simulink model "usb_servo_wzorzec"  (R2015a)
settings: Solver=ode4  StartTime=0.0  StopTime=300  FixedStep=0.01  RelTol=1e-3
Description:
  | Real-Time Van der Pol Simulation
  | 
  | This demonstration shows a real-time version of the Simulink Van der Pol
  | simulation demo. This model does not need any external signals, so it does
  | not need any data acquisition hardware or driver. This makes the model ideal
  | for first experiments with Real-Time Windows Target, without need to
  | worry about proper I/O hardware configuration.
  | 
  | How to run this demo:
  | 
  |   1. Build the model using Tools -> Real-Time Workshop -> Build Model.
  |   2. Connect to the real-time code using Simulation -> Connect to target.
  |   3. Start the real-time execution using Simulation -> Start real-time code.
settings Model: SimulationMode=external  CovSFcnEnable=off  ExtModeTrigDuration=6000  Creator=Houska  LastModifiedBy=Student
settings DataIOCC: SignalLoggingSaveFormat=ModelDataLogs  SaveOutput=off  SaveTime=off  SignalLoggingName=logsOut
settings OptimizationCC: ExpressionDepthLimit=2147483647  InitFltsAndDblsToZero=on
settings DebuggingCC: SaveWithParameterizedLinksMsg=none  UnderspecifiedInitializationDetection=Classic  MergeDetectMultiDrivingBlocksExec=none  SignalResolutionControl=TryResolveAllWithWarning  MultiTaskDSMMsg=warning  MultiTaskCondExecSysMsg=none  FcnCallInpInsideContextMsg=UseLocalSettings  StateNameClashWarn=warning
settings HardwareCC: ProdIntDivRoundTo=Zero  ProdEndianess=LittleEndian  ProdHWDeviceType=32-bit Real-Time Windows Target  TargetHWDeviceType=32-bit Generic  ProdEqTarget=off
settings RTWCC: SystemTargetFile=rtcon_servo_usb2.tlc  TemplateMakefile=servo_vc_usb2_x64.tmf  Description=servo (Visual C/C++)
settings STFCustomTargetCC: GenerateSampleERTMain=off  ModelReferenceCompliant=off  GeneratePreprocessorConditionals=Disable all  CombineOutputUpdateFcns=on  ERTCustomFileBanners=off  MatFileLogging=on  SupportNonInlinedSFcns=on  SupportVariableSizeSignals=off  MATLABClassNameForMDSCustomization=Simulink.SoftwareTarget.GRTCustomization  SystemTargetFile=rtcon_servo_usb2.tlc
settings GRTTargetCC: ModelReferenceCompliant=off  ParMdlRefBuildCompliant=off  CompOptLevelCompliant=off  ConcurrentExecutionCompliant=off  CPPClassGenCompliant=off  ExtMode=on  ExtModeMexFile=rtcon_ext_comm

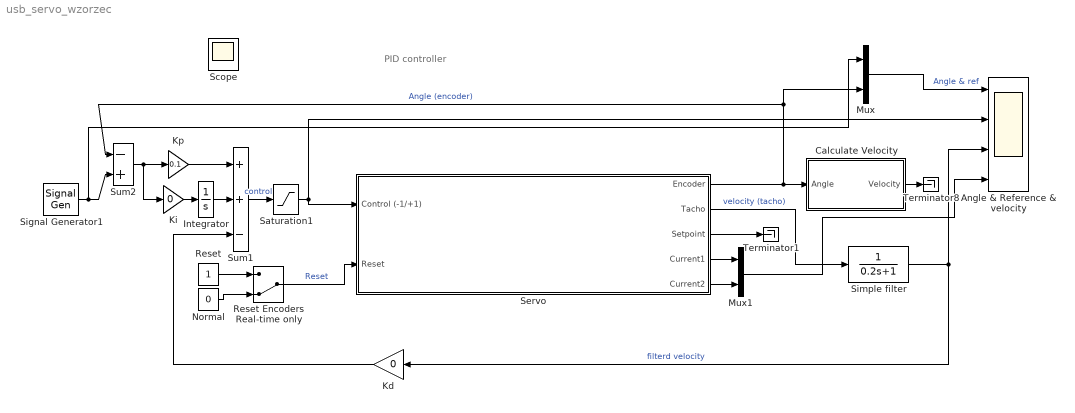
== system usb_servo_wzorzec ==
  note: PID controller
  Angle & Reference & velocity : Scope  NumInputPorts=4
      settings: TimeRange=30  YMin=-50~-0.6~-25~-10  YMax=60~0.6~45~8  SaveName=PD_C  MaxDataPoints=20000  Decimation=2
  Calculate Velocity : Subsystem
      mask Display: disp( 'rad-to-rad/s' )
  Integrator : Integrator
  Kd : Gain  Gain=0  SaturateOnIntegerOverflow=on  OutDataTypeStr=Inherit: Same as input  ParamDataTypeStr=Inherit: Same as input
  Ki : Gain  Gain=0  SaturateOnIntegerOverflow=on  OutDataTypeStr=Inherit: Same as input  ParamDataTypeStr=Inherit: Same as input
  Kp : Gain  Gain=0.1  SaturateOnIntegerOverflow=on  OutDataTypeStr=Inherit: Same as input  ParamDataTypeStr=Inherit: Same as input
  Mux : Mux  Inputs=2
  Mux1 : Mux  Inputs=2
  Normal : Constant  Value=0
  Reset : Constant
  Reset Encoders Real-time only : ManualSwitch  CurrentSetting=0
  Saturation1 : Saturate  UpperLimit=0.6  LowerLimit=-0.6
  Servo : Subsystem
      mask Display: image(imread('Servo.JPG'))
  Signal Generator1 : SignalGenerator  WaveForm=square  Amplitude=pi*25/2  Frequency=0.05
  Simple filter : TransferFcn  Denominator=[0.2 1]
  Sum1 : Sum  Inputs=++-  SaturateOnIntegerOverflow=on  InputSameDT=on  OutDataTypeStr=Inherit: Same as first input
  Sum2 : Sum  Inputs=-+  SaturateOnIntegerOverflow=on  InputSameDT=on  OutDataTypeStr=Inherit: Same as first input
  Terminator1 : Terminator
  Terminator8 : Terminator
  Scope : Scope
      settings: YMin=-5850  YMax=-5525
  wires:
  Mux/1 -> Angle & Reference & velocity/1  "Angle & ref"
  Servo/1(Encoder) -> Sum2/1, Mux/2, Calculate Velocity/1(Angle)  "Angle (encoder)"
  Reset Encoders Real-time only/1 -> Servo/2(Reset)  "Reset"
  Servo/2(Tacho) -> Simple filter/1  "velocity (tacho)"
  Normal/1 -> Reset Encoders Real-time only/2
  Reset/1 -> Reset Encoders Real-time only/1
  Servo/3(Setpoint) -> Terminator1/1
  Simple filter/1 -> Kd/1, Angle & Reference & velocity/3  "filterd velocity"
  Signal Generator1/1 -> Sum2/2, Mux/1
  Kp/1 -> Sum1/1
  Sum2/1 -> Kp/1, Ki/1
  Calculate Velocity/1(Velocity) -> Terminator8/1
  Kd/1 -> Sum1/3
  Saturation1/1 -> Angle & Reference & velocity/2, Servo/1(Control (-1/+1))
  Sum1/1 -> Saturation1/1  "control"
  Integrator/1 -> Sum1/2
  Ki/1 -> Integrator/1
  Servo/4(Current1) -> Mux1/1
  Servo/5(Current2) -> Mux1/2
  Mux1/1 -> Angle & Reference & velocity/4

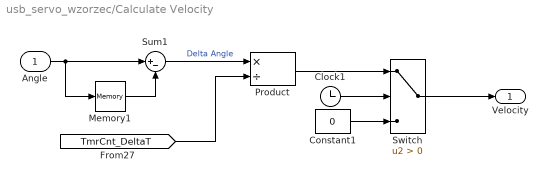
== system usb_servo_wzorzec/Calculate Velocity ==
  Angle : Inport
  Clock1 : Clock
  Constant1 : Constant  Value=0
  Memory1 : Memory
  Product : Product  Inputs=*/  SaturateOnIntegerOverflow=on  InputSameDT=on  OutDataTypeStr=Inherit: Same as first input
  Sum1 : Sum  Inputs=|+-  SaturateOnIntegerOverflow=on  InputSameDT=on  OutDataTypeStr=Inherit: Same as first input
  Switch : Switch  Criteria=u2 > Threshold  SaturateOnIntegerOverflow=on  InputSameDT=on
  Velocity : Outport
  wires:
  Switch/1 -> Velocity/1
  Constant1/1 -> Switch/3
  Clock1/1 -> Switch/2
  Product/1 -> Switch/1
  Sum1/1 -> Product/1  "Delta Angle"
  Angle/1 -> Memory1/1, Sum1/1
  Memory1/1 -> Sum1/2
  [TmrCnt_DeltaT] -> Product/2

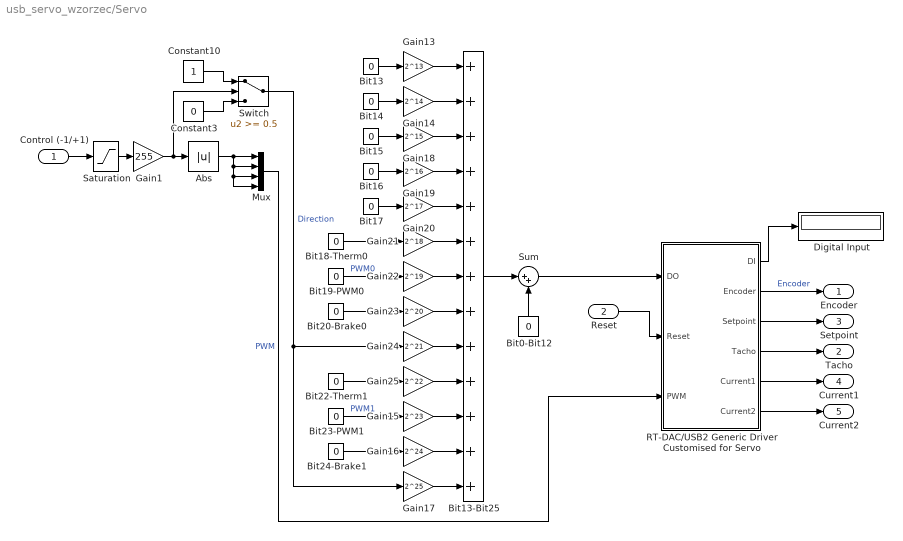
== system usb_servo_wzorzec/Servo ==
  Control (-1/+1) : Inport
  Reset : Inport  Port=2
  Abs : Abs  SaturateOnIntegerOverflow=on
  Bit0-Bit12 : Constant  Value=0
  Bit{13..17} (5 alike) : Constant  Value=0
  Bit13-Bit25 : Sum  Inputs=+++++++++++++  SaturateOnIntegerOverflow=on  InputSameDT=on  OutDataTypeStr=Inherit: Same as first input
  Bit18-Therm0 : Constant  Value=0
  Bit19-PWM0 : Constant  Value=0
  Bit20-Brake0 : Constant  Value=0
  Bit22-Therm1 : Constant  Value=0
  Bit23-PWM1 : Constant  Value=0
  Bit24-Brake1 : Constant  Value=0
  Constant10 : Constant
  Constant3 : Constant  Value=0
  Digital Input : Display
  Gain1 : Gain  Gain=255  SaturateOnIntegerOverflow=on  OutDataTypeStr=Inherit: Same as input  ParamDataTypeStr=Inherit: Same as input
  Gain13 : Gain  Gain=2^13  SaturateOnIntegerOverflow=on  OutDataTypeStr=Inherit: Same as input  ParamDataTypeStr=Inherit: Same as input
  Gain14 : Gain  Gain=2^14  SaturateOnIntegerOverflow=on  OutDataTypeStr=Inherit: Same as input  ParamDataTypeStr=Inherit: Same as input
  Gain15 : Gain  Gain=2^23  SaturateOnIntegerOverflow=on  OutDataTypeStr=Inherit: Same as input  ParamDataTypeStr=Inherit: Same as input
  Gain16 : Gain  Gain=2^24  SaturateOnIntegerOverflow=on  OutDataTypeStr=Inherit: Same as input  ParamDataTypeStr=Inherit: Same as input
  Gain17 : Gain  Gain=2^25  SaturateOnIntegerOverflow=on  OutDataTypeStr=Inherit: Same as input  ParamDataTypeStr=Inherit: Same as input
  Gain18 : Gain  Gain=2^15  SaturateOnIntegerOverflow=on  OutDataTypeStr=Inherit: Same as input  ParamDataTypeStr=Inherit: Same as input
  Gain19 : Gain  Gain=2^16  SaturateOnIntegerOverflow=on  OutDataTypeStr=Inherit: Same as input  ParamDataTypeStr=Inherit: Same as input
  Gain20 : Gain  Gain=2^17  SaturateOnIntegerOverflow=on  OutDataTypeStr=Inherit: Same as input  ParamDataTypeStr=Inherit: Same as input
  Gain21 : Gain  Gain=2^18  SaturateOnIntegerOverflow=on  OutDataTypeStr=Inherit: Same as input  ParamDataTypeStr=Inherit: Same as input
  Gain22 : Gain  Gain=2^19  SaturateOnIntegerOverflow=on  OutDataTypeStr=Inherit: Same as input  ParamDataTypeStr=Inherit: Same as input
  Gain23 : Gain  Gain=2^20  SaturateOnIntegerOverflow=on  OutDataTypeStr=Inherit: Same as input  ParamDataTypeStr=Inherit: Same as input
  Gain24 : Gain  Gain=2^21  SaturateOnIntegerOverflow=on  OutDataTypeStr=Inherit: Same as input  ParamDataTypeStr=Inherit: Same as input
  Gain25 : Gain  Gain=2^22  SaturateOnIntegerOverflow=on  OutDataTypeStr=Inherit: Same as input  ParamDataTypeStr=Inherit: Same as input
  Mux : Mux
  RT-DAC/USB2 Generic Driver Customised for Servo : Subsystem
      mask Display: disp('RT-DAC/USB2\n\nGeneric Driver\nVersion 2.1')
  Saturation : Saturate  UpperLimit=1  LowerLimit=-1
  Sum : Sum  Inputs=|++  SaturateOnIntegerOverflow=on  InputSameDT=on  OutDataTypeStr=Inherit: Same as first input
  Switch : Switch  Threshold=0.5  InputSameDT=on
  Encoder : Outport
  Tacho : Outport  Port=2
  Setpoint : Outport  Port=3
  Current1 : Outport  Port=4
  Current2 : Outport  Port=5
  wires:
  RT-DAC/USB2 Generic Driver Customised for Servo/4(Tacho) -> Tacho/1
  RT-DAC/USB2 Generic Driver Customised for Servo/3(Setpoint) -> Setpoint/1
  RT-DAC/USB2 Generic Driver Customised for Servo/2(Encoder) -> Encoder/1  "Encoder"
  Mux/1 -> RT-DAC/USB2 Generic Driver Customised for Servo/3(PWM)  "PWM"
  Switch/1 -> Gain17/1, Gain24/1  "Direction"
  Abs/1 -> Mux/4, Mux/3, Mux/2, Mux/1
  Constant3/1 -> Switch/3
  Constant10/1 -> Switch/1
  Gain1/1 -> Switch/2, Abs/1
  Saturation/1 -> Gain1/1
  Control (-1/+1)/1 -> Saturation/1
  Reset/1 -> RT-DAC/USB2 Generic Driver Customised for Servo/2(Reset)
  Bit24-Brake1/1 -> Gain16/1
  Bit23-PWM1/1 -> Gain15/1  "PWM1"
  Bit22-Therm1/1 -> Gain25/1
  Bit13-Bit25/1 -> Sum/1
  Sum/1 -> RT-DAC/USB2 Generic Driver Customised for Servo/1(DO)
  Gain17/1 -> Bit13-Bit25/13
  Gain16/1 -> Bit13-Bit25/12
  Gain15/1 -> Bit13-Bit25/11
  Gain25/1 -> Bit13-Bit25/10
  Gain24/1 -> Bit13-Bit25/9
  Gain23/1 -> Bit13-Bit25/8
  Gain22/1 -> Bit13-Bit25/7
  Gain21/1 -> Bit13-Bit25/6
  Gain20/1 -> Bit13-Bit25/5
  Gain19/1 -> Bit13-Bit25/4
  Gain18/1 -> Bit13-Bit25/3
  Gain14/1 -> Bit13-Bit25/2
  Gain13/1 -> Bit13-Bit25/1
  Bit0-Bit12/1 -> Sum/2
  RT-DAC/USB2 Generic Driver Customised for Servo/1(DI) -> Digital Input/1
  Bit20-Brake0/1 -> Gain23/1
  Bit19-PWM0/1 -> Gain22/1  "PWM0"
  Bit18-Therm0/1 -> Gain21/1
  Bit17/1 -> Gain20/1
  Bit16/1 -> Gain19/1
  Bit15/1 -> Gain18/1
  Bit14/1 -> Gain14/1
  Bit13/1 -> Gain13/1
  RT-DAC/USB2 Generic Driver Customised for Servo/6(Current2) -> Current2/1
  RT-DAC/USB2 Generic Driver Customised for Servo/5(Current1) -> Current1/1

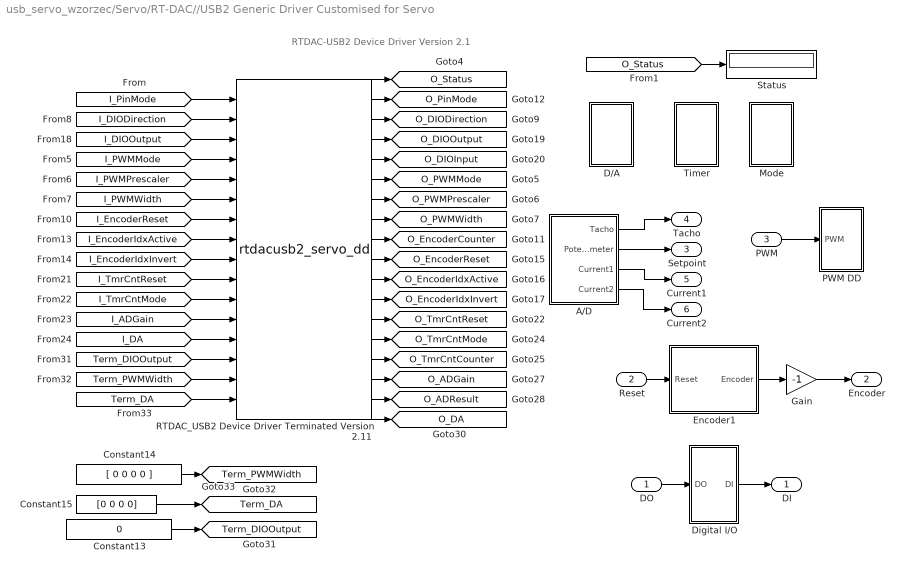
== system usb_servo_wzorzec/Servo/RT-DAC//USB2 Generic Driver Customised for Servo ==
  note: RTDAC-USB2 Device Driver
      | Version 2.1
  DO : Inport
  Reset : Inport  Port=2
  PWM : Inport  Port=3
  A/D : Subsystem
  Constant13 : Constant  Value=0
  Constant14 : Constant  Value=[ 0 0 0 0 ]
  Constant15 : Constant  Value=[0 0 0 0]
  D/A : Subsystem
  Digital I/O : Subsystem
  Encoder1 : Subsystem
  Gain : Gain  Gain=-1
  Mode : Subsystem
  PWM DD : Subsystem
  RTDAC_USB2 Device Driver Terminated Version 2.11 : S-Function  FunctionName=rtdacusb2_servo_dd  Parameters=0.01
  Status : Display
  Timer : Subsystem
  DI : Outport
  Encoder : Outport  Port=2
  Setpoint : Outport  Port=3
  Tacho : Outport  Port=4
  Current1 : Outport  Port=5
  Current2 : Outport  Port=6
  tag scope: O_ADGain=global, O_ADResult=global, O_DA=global, O_DIODirection=global, O_DIOInput=global, O_DIOOutput=global, O_EncoderCounter=global, O_EncoderIdxActive=global, O_EncoderIdxInvert=global, O_EncoderReset=global, O_PWMMode=global, O_PWMPrescaler=global, O_PWMWidth=global, O_PinMode=global, O_Status=global, O_TmrCntCounter=global, O_TmrCntMode=global, O_TmrCntReset=global, Term_DA=global, Term_DIOOutput=global, Term_PWMWidth=global
  wires:
  Constant14/1 -> [Term_PWMWidth]
  [Term_DA] -> RTDAC_USB2 Device Driver Terminated Version 2.11/16
  [Term_PWMWidth] -> RTDAC_USB2 Device Driver Terminated Version 2.11/15
  [Term_DIOOutput] -> RTDAC_USB2 Device Driver Terminated Version 2.11/14
  Constant13/1 -> [Term_DIOOutput]
  Constant15/1 -> [Term_DA]
  A/D/1(Tacho) -> Tacho/1
  A/D/2(Potentiometer) -> Setpoint/1
  Reset/1 -> Encoder1/1(Reset)
  Digital I/O/1(DI) -> DI/1
  DO/1 -> Digital I/O/1(DO)
  Encoder1/1(Encoder) -> Gain/1
  RTDAC_USB2 Device Driver Terminated Version 2.11/5 -> [O_DIOInput]
  RTDAC_USB2 Device Driver Terminated Version 2.11/4 -> [O_DIOOutput]
  [I_DIOOutput] -> RTDAC_USB2 Device Driver Terminated Version 2.11/3
  RTDAC_USB2 Device Driver Terminated Version 2.11/12 -> [O_EncoderIdxInvert]
  RTDAC_USB2 Device Driver Terminated Version 2.11/11 -> [O_EncoderIdxActive]
  RTDAC_USB2 Device Driver Terminated Version 2.11/10 -> [O_EncoderReset]
  [I_EncoderIdxInvert] -> RTDAC_USB2 Device Driver Terminated Version 2.11/9
  [I_EncoderIdxActive] -> RTDAC_USB2 Device Driver Terminated Version 2.11/8
  RTDAC_USB2 Device Driver Terminated Version 2.11/2 -> [O_PinMode]
  RTDAC_USB2 Device Driver Terminated Version 2.11/3 -> [O_DIODirection]
  RTDAC_USB2 Device Driver Terminated Version 2.11/9 -> [O_EncoderCounter]
  [I_EncoderReset] -> RTDAC_USB2 Device Driver Terminated Version 2.11/7
  [I_DIODirection] -> RTDAC_USB2 Device Driver Terminated Version 2.11/2
  [I_PWMWidth] -> RTDAC_USB2 Device Driver Terminated Version 2.11/6
  [I_PWMPrescaler] -> RTDAC_USB2 Device Driver Terminated Version 2.11/5
  [I_PWMMode] -> RTDAC_USB2 Device Driver Terminated Version 2.11/4
  RTDAC_USB2 Device Driver Terminated Version 2.11/8 -> [O_PWMWidth]
  RTDAC_USB2 Device Driver Terminated Version 2.11/7 -> [O_PWMPrescaler]
  RTDAC_USB2 Device Driver Terminated Version 2.11/6 -> [O_PWMMode]
  [O_Status] -> Status/1
  RTDAC_USB2 Device Driver Terminated Version 2.11/1 -> [O_Status]
  PWM/1 -> PWM DD/1(PWM)
  [I_PinMode] -> RTDAC_USB2 Device Driver Terminated Version 2.11/1
  [I_TmrCntReset] -> RTDAC_USB2 Device Driver Terminated Version 2.11/10
  [I_ADGain] -> RTDAC_USB2 Device Driver Terminated Version 2.11/12
  [I_TmrCntMode] -> RTDAC_USB2 Device Driver Terminated Version 2.11/11
  [I_DA] -> RTDAC_USB2 Device Driver Terminated Version 2.11/13
  RTDAC_USB2 Device Driver Terminated Version 2.11/13 -> [O_TmrCntReset]
  RTDAC_USB2 Device Driver Terminated Version 2.11/14 -> [O_TmrCntMode]
  RTDAC_USB2 Device Driver Terminated Version 2.11/15 -> [O_TmrCntCounter]
  RTDAC_USB2 Device Driver Terminated Version 2.11/16 -> [O_ADGain]
  RTDAC_USB2 Device Driver Terminated Version 2.11/17 -> [O_ADResult]
  RTDAC_USB2 Device Driver Terminated Version 2.11/18 -> [O_DA]
  A/D/3(Current1) -> Current1/1
  A/D/4(Current2) -> Current2/1
  Gain/1 -> Encoder/1

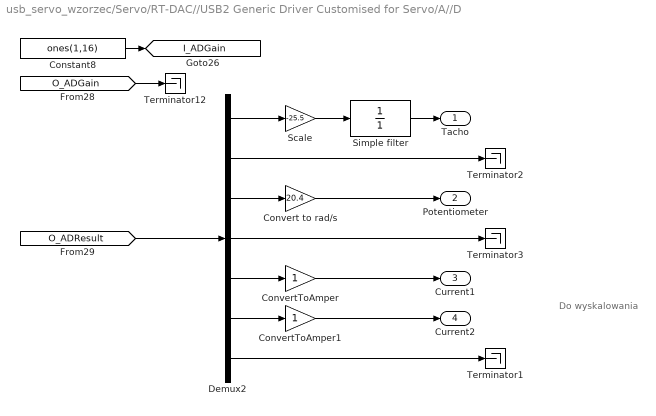
== system usb_servo_wzorzec/Servo/RT-DAC//USB2 Generic Driver Customised for Servo/A//D ==
  note: Do wyskalowania
  Constant8 : Constant  Value=ones(1,16)
  Convert to rad/s : Gain  Gain=20.4  OutDataTypeStr=Inherit: Same as input  ParamDataTypeStr=Inherit: Same as input
  ConvertToAmper : Gain  OutDataTypeStr=Inherit: Same as input  ParamDataTypeStr=Inherit: Same as input
  ConvertToAmper1 : Gain  OutDataTypeStr=Inherit: Same as input  ParamDataTypeStr=Inherit: Same as input
  Demux2 : Demux  Outputs=[1 1 1 1 1 1 10]
  Scale : Gain  Gain=-25.5  OutDataTypeStr=Inherit: Same as input  ParamDataTypeStr=Inherit: Same as input
  Simple filter : TransferFcn  Denominator=[0.0 1]
  Terminator{1..3,12} (4 alike) : Terminator
  Tacho : Outport  InitialOutput=0
  Potentiometer : Outport  Port=2  InitialOutput=0
  Current1 : Outport  Port=3  InitialOutput=0
  Current2 : Outport  Port=4  InitialOutput=0
  tag scope: I_ADGain=global
  wires:
  Scale/1 -> Simple filter/1
  Demux2/7 -> Terminator1/1
  Simple filter/1 -> Tacho/1
  Convert to rad/s/1 -> Potentiometer/1
  Demux2/1 -> Scale/1
  Constant8/1 -> [I_ADGain]
  [O_ADGain] -> Terminator12/1
  [O_ADResult] -> Demux2/1
  Demux2/3 -> Convert to rad/s/1
  Demux2/2 -> Terminator2/1
  Demux2/5 -> ConvertToAmper/1
  Demux2/6 -> ConvertToAmper1/1
  Demux2/4 -> Terminator3/1
  ConvertToAmper/1 -> Current1/1
  ConvertToAmper1/1 -> Current2/1

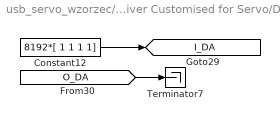
== system usb_servo_wzorzec/Servo/RT-DAC//USB2 Generic Driver Customised for Servo/D//A ==
  Constant12 : Constant  Value=8192*[ 1 1 1 1]
  Terminator7 : Terminator
  tag scope: I_DA=global
  wires:
  [O_DA] -> Terminator7/1
  Constant12/1 -> [I_DA]

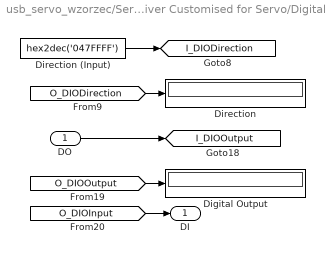
== system usb_servo_wzorzec/Servo/RT-DAC//USB2 Generic Driver Customised for Servo/Digital I//O ==
  DO : Inport
  Digital Output : Display
  Direction : Display
  Direction (Input) : Constant  Value=hex2dec('047FFFF')
  DI : Outport
  tag scope: I_DIODirection=global, I_DIOOutput=global
  wires:
  [O_DIOInput] -> DI/1
  [O_DIOOutput] -> Digital Output/1
  DO/1 -> [I_DIOOutput]
  [O_DIODirection] -> Direction/1
  Direction (Input)/1 -> [I_DIODirection]

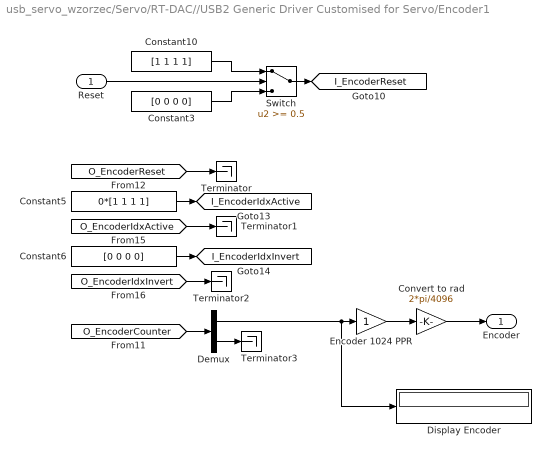
== system usb_servo_wzorzec/Servo/RT-DAC//USB2 Generic Driver Customised for Servo/Encoder1 ==
  Reset : Inport
  Constant10 : Constant  Value=[1 1 1 1]
  Constant3 : Constant  Value=[0 0 0 0]
  Constant5 : Constant  Value=0*[1 1 1 1]
  Constant6 : Constant  Value=[0 0 0 0]
  Convert to rad : Gain  Gain=2*pi/4096  SaturateOnIntegerOverflow=on  OutDataTypeStr=Inherit: Same as input  ParamDataTypeStr=Inherit: Same as input
  Demux : Demux  Outputs=[1 3]
  Display Encoder : Display
  Encoder 1024 PPR : Gain  SaturateOnIntegerOverflow=on  OutDataTypeStr=Inherit: Same as input  ParamDataTypeStr=Inherit: Same as input
  Switch : Switch  Threshold=0.5  InputSameDT=on
  Terminator{,1..3} (4 alike) : Terminator
  Encoder : Outport
  tag scope: I_EncoderIdxActive=global, I_EncoderIdxInvert=global, I_EncoderReset=global
  wires:
  Convert to rad/1 -> Encoder/1
  Demux/1 -> Encoder 1024 PPR/1, Display Encoder/1
  Encoder 1024 PPR/1 -> Convert to rad/1
  Reset/1 -> Switch/2
  Constant3/1 -> Switch/3
  Constant10/1 -> Switch/1
  Switch/1 -> [I_EncoderReset]
  Demux/2 -> Terminator3/1
  [O_EncoderIdxInvert] -> Terminator2/1
  [O_EncoderIdxActive] -> Terminator1/1
  Constant6/1 -> [I_EncoderIdxInvert]
  Constant5/1 -> [I_EncoderIdxActive]
  [O_EncoderReset] -> Terminator/1
  [O_EncoderCounter] -> Demux/1

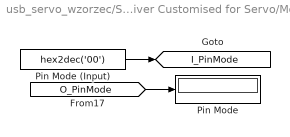
== system usb_servo_wzorzec/Servo/RT-DAC//USB2 Generic Driver Customised for Servo/Mode ==
  Pin Mode : Display
  Pin Mode (Input) : Constant  Value=hex2dec('00')
  tag scope: I_PinMode=global
  wires:
  Pin Mode (Input)/1 -> [I_PinMode]
  [O_PinMode] -> Pin Mode/1

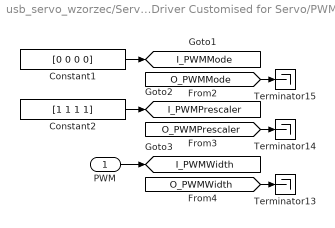
== system usb_servo_wzorzec/Servo/RT-DAC//USB2 Generic Driver Customised for Servo/PWM DD ==
  PWM : Inport
  Constant1 : Constant  Value=[0 0 0 0]
  Constant2 : Constant  Value=[1 1 1 1]
  Terminator13 : Terminator
  Terminator14 : Terminator
  Terminator15 : Terminator
  tag scope: I_PWMMode=global, I_PWMPrescaler=global, I_PWMWidth=global
  wires:
  PWM/1 -> [I_PWMWidth]
  [O_PWMWidth] -> Terminator13/1
  [O_PWMPrescaler] -> Terminator14/1
  [O_PWMMode] -> Terminator15/1
  Constant2/1 -> [I_PWMPrescaler]
  Constant1/1 -> [I_PWMMode]

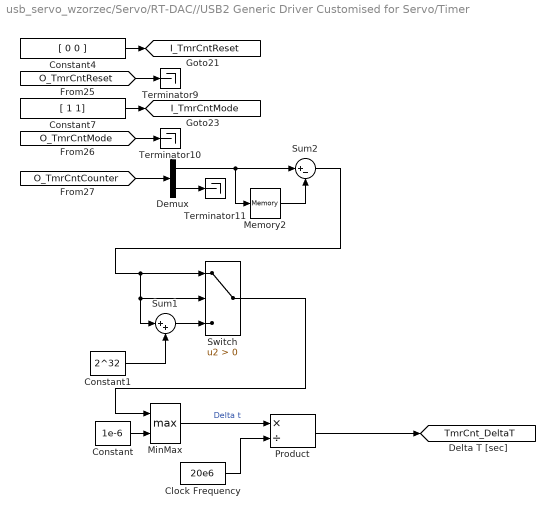
== system usb_servo_wzorzec/Servo/RT-DAC//USB2 Generic Driver Customised for Servo/Timer ==
  Clock Frequency : Constant  Value=20e6
  Constant : Constant  Value=1e-6
  Constant1 : Constant  Value=2^32
  Constant4 : Constant  Value=[ 0 0 ]
  Constant7 : Constant  Value=[ 1 1]
  Demux : Demux  Outputs=2
  Memory2 : Memory
  MinMax : MinMax  Function=max  Inputs=2  SaturateOnIntegerOverflow=on  InputSameDT=on
  Product : Product  Inputs=*/  SaturateOnIntegerOverflow=on  OutDataTypeStr=Inherit: Same as first input
  Sum1 : Sum  Inputs=|++  SaturateOnIntegerOverflow=on  InputSameDT=on  OutDataTypeStr=Inherit: Same as first input
  Sum2 : Sum  Inputs=|+-  SaturateOnIntegerOverflow=on  InputSameDT=on  OutDataTypeStr=Inherit: Same as first input
  Switch : Switch  Criteria=u2 > Threshold  SaturateOnIntegerOverflow=on  InputSameDT=on
  Terminator10 : Terminator
  Terminator11 : Terminator
  Terminator9 : Terminator
  tag scope: I_TmrCntMode=global, I_TmrCntReset=global, TmrCnt_DeltaT=global
  wires:
  Demux/2 -> Terminator11/1
  Demux/1 -> Sum2/1, Memory2/1
  Switch/1 -> MinMax/1
  Constant1/1 -> Sum1/2
  Sum1/1 -> Switch/3
  Sum2/1 -> Sum1/1, Switch/2, Switch/1
  Clock Frequency/1 -> Product/2
  MinMax/1 -> Product/1  "Delta t"
  Product/1 -> [TmrCnt_DeltaT]
  [O_TmrCntCounter] -> Demux/1
  Memory2/1 -> Sum2/2
  Constant/1 -> MinMax/2
  Constant4/1 -> [I_TmrCntReset]
  [O_TmrCntReset] -> Terminator9/1
  Constant7/1 -> [I_TmrCntMode]
  [O_TmrCntMode] -> Terminator10/1
